simulink model "Robot_2_links"  (Simulink 8.7)
settings: Solver=ode45  StartTime=0.0  StopTime=10  RelTol=1e-3
values from neighbouring files (symbols this model uses):
  i = 100    [Robot_2_links_params.m]
  Jrot = [0.0037 0.0008]    [Robot_2_links_params.m]
  Ki = [1.563 3.125]    [Robot_2_links_params.m]
  Koss = [1 1]    [Robot_2_links_params.m]
  Kp = [800 350]    [Robot_2_links_params.m]
  Kpp = [0.05 0.05]    [Robot_2_links_params.m]
  l1 = 0.6    [Robot_2_links_params.m]
  l2 = 0.4    [Robot_2_links_params.m]
  m1 = 15    [Robot_2_links_params.m]
  m2 = m2link+m2load    (= 25)    [Robot_2_links_params.m]
  q1inp = 1    [Robot_2_links_params.m]
  q2inp = 1    [Robot_2_links_params.m]
  switch_coord = 0    [Robot_2_links_params.m]
  T = [0.02 0.01]    [Robot_2_links_params.m]
  xinp = 0.2    [Robot_2_links_params.m]
  yinp = 0.3    [Robot_2_links_params.m]
undefined symbols (not defined in the file or in its folder): sfunxy
settings Model: Creator=Student  LastModifiedBy=Руслан
settings DataIOCC: LimitDataPoints=off  SaveFormat=StructureWithTime  SignalLoggingSaveFormat=ModelDataLogs
settings DebuggingCC: UnderspecifiedInitializationDetection=Simplified  MergeDetectMultiDrivingBlocksExec=error  FcnCallInpInsideContextMsg=EnableAllAsWarning
settings HardwareCC: ProdIntDivRoundTo=Zero  ProdEndianess=LittleEndian  ProdHWDeviceType=Specified
settings GRTTargetCC: GeneratePreprocessorConditionals=Use local settings  CombineOutputUpdateFcns=off  GRTInterface=on
settings ConfigComp: CovModelRefEnable=off

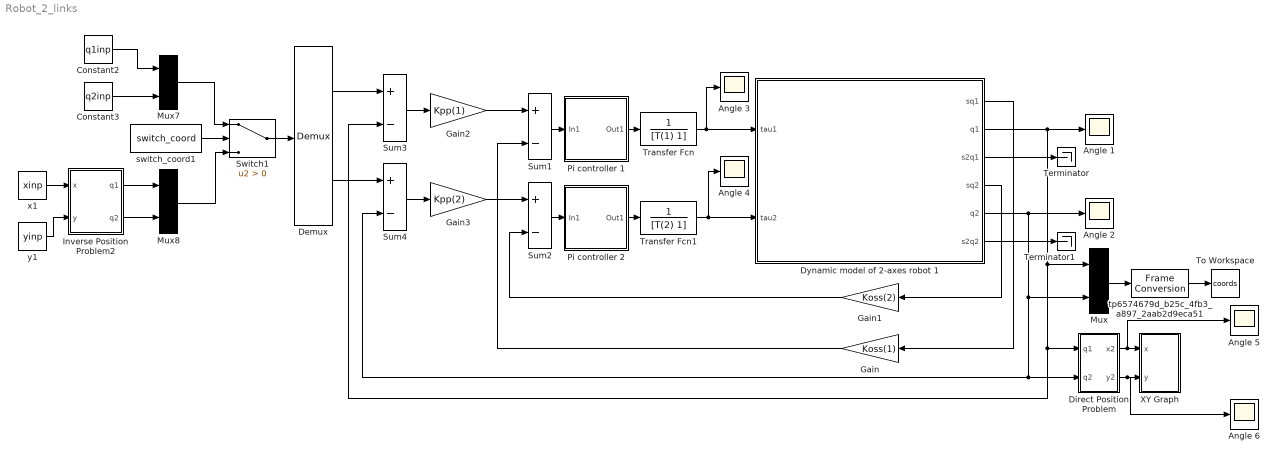
== system Robot_2_links ==
  Angle {1..6} (6 alike) : Scope
  Constant2 : Constant  Value=q1inp
  Constant3 : Constant  Value=q2inp
  Demux : Demux  Outputs=2
  Direct Position Problem : Subsystem
  Dynamic model of 2-axes robot 1 : Subsystem
  Gain : Gain  Gain=Koss(1)
  Gain1 : Gain  Gain=Koss(2)
  Gain2 : Gain  Gain=Kpp(1)
  Gain3 : Gain  Gain=Kpp(2)
  Inverse Position Problem2 : Subsystem
  Mux : Mux  Inputs=2
  Mux7 : Mux  Inputs=2
  Mux8 : Mux  Inputs=2
  Pi controller 1 : Subsystem
  Pi controller 2 : Subsystem
  Sum{1..4} (4 alike) : Sum  Inputs=+-
  Switch1 : Switch  Criteria=u2 > Threshold
  Terminator : Terminator
  Terminator1 : Terminator
  To Workspace : ToWorkspace  VariableName=coords  SampleTime=-1
  Transfer Fcn : TransferFcn  Denominator=[T(1) 1]
  Transfer Fcn1 : TransferFcn  Denominator=[T(2) 1]
  XY Graph : Subsystem  LoadFcn=sfunxy([],[],[],'LoadBlock')  StartFcn=sfunxy([],[],[],'Start')  StopFcn=sfunxy([],[],[],'Stop')  TreatAsAtomicUnit=on  SimViewingDevice=on  mask(XY scope.){xmin=-1, xmax=1, ymin=-1, ymax=1, st=-1}
      mask prompts: xmin "Simulink:masks:xmin_MP"; xmax "Simulink:masks:xmax_MP"; ymin "Simulink:masks:ymin_MP"; ymax "Simulink:masks:ymax_MP"; st "Simulink:masks:SampleTime_MP"
      mask help: Simulink:masks:XYScope_MD
      settings: CopyFcn=sfunxy([],[],[],'CopyBlock')  DeleteFcn=sfunxy([],[],[],'DeleteBlock')  NameChangeFcn=sfunxy([],[],[],'NameChange')
      mask Help: This block can be used to explore limit cycles. Look at the m-file sfunxy.m to see how it works.
      mask Display: plot([.05 .95 .95 .05 .05],[.45 .45 .95 .95 .45], 0.5+cos(0:0.1:2*pi)*0.3,0.7+sin(0:0.1:2*pi)*0.2)
  switch_coord1 : Constant  Value=switch_coord
  tp6574679d_b25c_4fb3_a897_2aab2d9eca51 : FrameConversion  InheritSamplingMode=off  OutFrame=Sample-based
  x1 : Constant  Value=xinp
  y1 : Constant  Value=yinp
  wires:
  Pi controller 1/1(Out1) -> Transfer Fcn/1
  Pi controller 2/1(Out1) -> Transfer Fcn1/1
  Dynamic model of 2-axes robot 1/5(q2) -> Sum4/2, Direct Position Problem/2(q2), Mux/2, Angle 2/1
  Sum2/1 -> Pi controller 2/1(In1)
  Sum1/1 -> Pi controller 1/1(In1)
  Gain/1 -> Sum1/2
  Gain1/1 -> Sum2/2
  Gain2/1 -> Sum1/1
  Gain3/1 -> Sum2/1
  Sum3/1 -> Gain2/1
  Sum4/1 -> Gain3/1
  Dynamic model of 2-axes robot 1/4(sq2) -> Gain1/1
  Dynamic model of 2-axes robot 1/1(sq1) -> Gain/1
  Dynamic model of 2-axes robot 1/2(q1) -> Angle 1/1, Direct Position Problem/1(q1), Sum3/2, Mux/1
  Direct Position Problem/1(x2) -> Angle 5/1, XY Graph/1(x)
  Direct Position Problem/2(y2) -> Angle 6/1, XY Graph/2(y)
  Demux/1 -> Sum3/1
  Switch1/1 -> Demux/1
  Demux/2 -> Sum4/1
  Dynamic model of 2-axes robot 1/3(s2q1) -> Terminator/1
  Dynamic model of 2-axes robot 1/6(s2q2) -> Terminator1/1
  Transfer Fcn/1 -> Dynamic model of 2-axes robot 1/1(tau1), Angle 3/1
  Transfer Fcn1/1 -> Dynamic model of 2-axes robot 1/2(tau2), Angle 4/1
  Constant2/1 -> Mux7/1
  Mux8/1 -> Switch1/3
  Constant3/1 -> Mux7/2
  Inverse Position Problem2/1(q1) -> Mux8/1
  Inverse Position Problem2/2(q2) -> Mux8/2
  y1/1 -> Inverse Position Problem2/2(y)
  x1/1 -> Inverse Position Problem2/1(x)
  switch_coord1/1 -> Switch1/2
  Mux7/1 -> Switch1/1
  Mux/1 -> tp6574679d_b25c_4fb3_a897_2aab2d9eca51/1
  tp6574679d_b25c_4fb3_a897_2aab2d9eca51/1 -> To Workspace/1

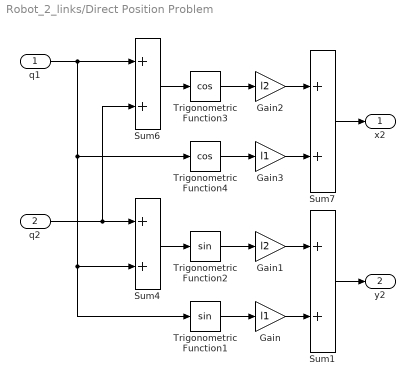
== system Robot_2_links/Direct Position Problem ==
  q1 : Inport
  q2 : Inport  Port=2
  Gain : Gain  Gain=l1
  Gain1 : Gain  Gain=l2
  Gain2 : Gain  Gain=l2
  Gain3 : Gain  Gain=l1
  Sum{1,4,6..7} (4 alike) : Sum
  Trigonometric Function1 : Trigonometry
  Trigonometric Function2 : Trigonometry
  Trigonometric Function3 : Trigonometry  Operator=cos
  Trigonometric Function4 : Trigonometry  Operator=cos
  x2 : Outport
  y2 : Outport  Port=2
  wires:
  Trigonometric Function1/1 -> Gain/1
  Sum4/1 -> Trigonometric Function2/1
  Gain3/1 -> Sum7/2
  Sum1/1 -> y2/1
  Trigonometric Function2/1 -> Gain1/1
  Sum6/1 -> Trigonometric Function3/1
  Sum7/1 -> x2/1
  Trigonometric Function3/1 -> Gain2/1
  Gain2/1 -> Sum7/1
  Trigonometric Function4/1 -> Gain3/1
  q2/1 -> Sum4/1, Sum6/2
  q1/1 -> Trigonometric Function4/1, Trigonometric Function1/1, Sum4/2, Sum6/1
  Gain1/1 -> Sum1/1
  Gain/1 -> Sum1/2

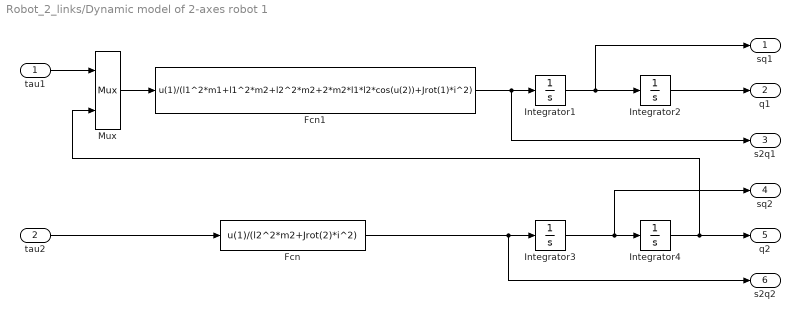
== system Robot_2_links/Dynamic model of 2-axes robot 1 ==
  tau1 : Inport
  tau2 : Inport  Port=2
  Fcn : Fcn  Expr=u(1)/(l2^2*m2+Jrot(2)*i^2)
  Fcn1 : Fcn  Expr=u(1)/(l1^2*m1+l1^2*m2+l2^2*m2+2*m2*l1*l2*cos(u(2))+Jrot(1)*i^2)
  Integrator1 : Integrator
  Integrator2 : Integrator  UpperSaturationLimit=3.142  LowerSaturationLimit=-1.571
  Integrator3 : Integrator
  Integrator4 : Integrator  UpperSaturationLimit=3.142  LowerSaturationLimit=-1.571
  Mux : Mux  Inputs=2
  sq1 : Outport
  q1 : Outport  Port=2
  s2q1 : Outport  Port=3
  sq2 : Outport  Port=4
  q2 : Outport  Port=5
  s2q2 : Outport  Port=6
  wires:
  Fcn1/1 -> s2q1/1, Integrator1/1
  Fcn/1 -> s2q2/1, Integrator3/1
  Integrator2/1 -> q1/1
  Integrator4/1 -> Mux/2, q2/1
  Integrator1/1 -> sq1/1, Integrator2/1
  Integrator3/1 -> sq2/1, Integrator4/1
  tau2/1 -> Fcn/1
  Mux/1 -> Fcn1/1
  tau1/1 -> Mux/1

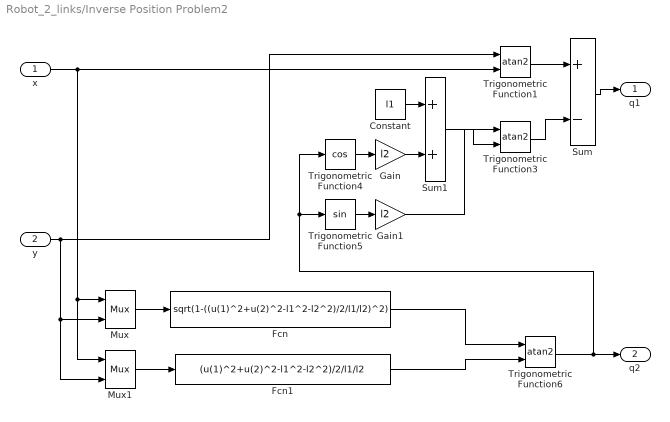
== system Robot_2_links/Inverse Position Problem2 ==
  x : Inport
  y : Inport  Port=2
  Constant : Constant  Value=l1
  Fcn : Fcn  Expr=sqrt(1-((u(1)^2+u(2)^2-l1^2-l2^2)/2/l1/l2)^2)
  Fcn1 : Fcn  Expr=(u(1)^2+u(2)^2-l1^2-l2^2)/2/l1/l2
  Gain : Gain  Gain=l2
  Gain1 : Gain  Gain=l2
  Mux : Mux  Inputs=2
  Mux1 : Mux  Inputs=2
  Sum : Sum  Inputs=+-
  Sum1 : Sum
  Trigonometric Function1 : Trigonometry  Operator=atan2
  Trigonometric Function3 : Trigonometry  Operator=atan2
  Trigonometric Function4 : Trigonometry  Operator=cos
  Trigonometric Function5 : Trigonometry
  Trigonometric Function6 : Trigonometry  Operator=atan2
  q1 : Outport
  q2 : Outport  Port=2
  wires:
  Sum/1 -> q1/1
  Trigonometric Function1/1 -> Sum/1
  y/1 -> Mux1/2, Mux/2, Trigonometric Function1/1
  x/1 -> Mux1/1, Mux/1, Trigonometric Function1/2
  Trigonometric Function3/1 -> Sum/2
  Constant/1 -> Sum1/1
  Trigonometric Function4/1 -> Gain/1
  Gain/1 -> Sum1/2
  Sum1/1 -> Trigonometric Function3/2
  Trigonometric Function5/1 -> Gain1/1
  Gain1/1 -> Trigonometric Function3/1
  Trigonometric Function6/1 -> Trigonometric Function4/1, Trigonometric Function5/1, q2/1
  Mux/1 -> Fcn/1
  Fcn/1 -> Trigonometric Function6/1
  Mux1/1 -> Fcn1/1
  Fcn1/1 -> Trigonometric Function6/2

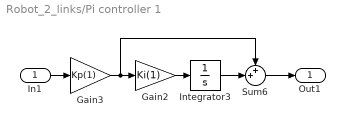
== system Robot_2_links/Pi controller 1 ==
  In1 : Inport
  Gain2 : Gain  Gain=Ki(1)
  Gain3 : Gain  Gain=Kp(1)
  Integrator3 : Integrator
  Sum6 : Sum  Inputs=++|
  Out1 : Outport
  wires:
  Integrator3/1 -> Sum6/2
  Gain3/1 -> Sum6/1, Gain2/1
  Gain2/1 -> Integrator3/1
  Sum6/1 -> Out1/1
  In1/1 -> Gain3/1

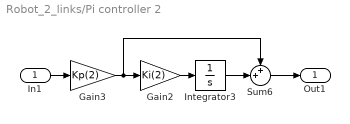
== system Robot_2_links/Pi controller 2 ==
  In1 : Inport
  Gain2 : Gain  Gain=Ki(2)
  Gain3 : Gain  Gain=Kp(2)
  Integrator3 : Integrator
  Sum6 : Sum  Inputs=++|
  Out1 : Outport
  wires:
  Integrator3/1 -> Sum6/2
  Gain3/1 -> Gain2/1, Sum6/1
  Gain2/1 -> Integrator3/1
  Sum6/1 -> Out1/1
  In1/1 -> Gain3/1

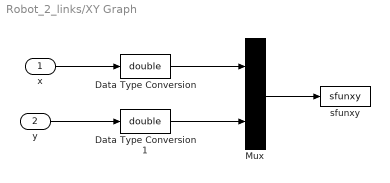
== system Robot_2_links/XY Graph ==
  x : Inport
  y : Inport  Port=2
  Data Type Conversion : DataTypeConversion  DisableCoverage=on  OutDataTypeStr=double
  Data Type Conversion1 : DataTypeConversion  DisableCoverage=on  OutDataTypeStr=double
  Mux : Mux  Inputs=2
  sfunxy : S-Function  DisableCoverage=on  FunctionName=sfunxy  Parameters=[xmin xmax ymin ymax], st  SFunctionDeploymentMode=off  EnableBusSupport=off
  wires:
  Data Type Conversion1/1 -> Mux/2
  Data Type Conversion/1 -> Mux/1
  y/1 -> Data Type Conversion1/1
  x/1 -> Data Type Conversion/1
  Mux/1 -> sfunxy/1
